simulink model "Assignment7"  (R2019a)
settings: Solver=FixedStepDiscrete  StartTime=0.0  StopTime=40  FixedStep=1  RelTol=1e-3
libraries: simulink x3
settings Model: Creator=Acer  LastModifiedBy=Acer

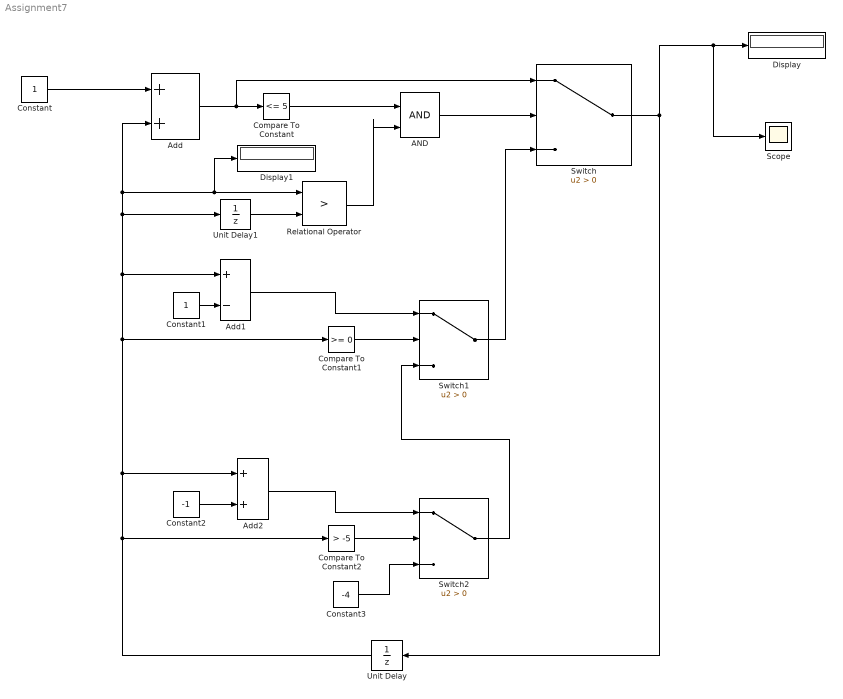
== system Assignment7 ==
  AND : Logic  IconShape=distinctive  AllPortsSameDT=off  OutDataTypeStr=boolean
  Add : Sum
  Add1 : Sum  Inputs=+-
  Add2 : Sum
  Compare To Constant : simulink/Logic and Bit Operations/Compare To Constant  relop=<=  const=5  OutDataTypeStr=boolean
  Compare To Constant1 : simulink/Logic and Bit Operations/Compare To Constant  relop=>=  const=0  OutDataTypeStr=boolean
  Compare To Constant2 : simulink/Logic and Bit Operations/Compare To Constant  relop=>  const=-5  OutDataTypeStr=boolean
  Constant : Constant
  Constant1 : Constant
  Constant2 : Constant  Value=-1
  Constant3 : Constant  Value=-4
  Display : Display
  Display1 : Display
  Relational Operator : RelationalOperator  Operator=>  OutDataTypeStr=boolean  RndMeth=Simplest
  Scope : Scope
  Switch : Switch  Criteria=u2 > Threshold
  Switch1 : Switch  Criteria=u2 > Threshold
  Switch2 : Switch  Criteria=u2 > Threshold
  Unit Delay : UnitDelay  InitialCondition=-1  SampleTime=-1  HasFrameUpgradeWarning=on
  Unit Delay1 : UnitDelay  InitialCondition=-2  SampleTime=-1  HasFrameUpgradeWarning=on
  wires:
  Constant/1 -> Add/1
  Add/1 -> Switch/1, Compare To Constant/1
  AND/1 -> Switch/2
  Compare To Constant/1 -> AND/1
  Switch/1 -> Scope/1, Display/1, Unit Delay/1
  Unit Delay/1 -> Add/2, Display1/1, Relational Operator/1, Unit Delay1/1, Add1/1, Compare To Constant1/1, Add2/1, Compare To Constant2/1
  Relational Operator/1 -> AND/2
  Unit Delay1/1 -> Relational Operator/2
  Compare To Constant1/1 -> Switch1/2
  Switch1/1 -> Switch/3
  Constant1/1 -> Add1/2
  Add1/1 -> Switch1/1
  Add2/1 -> Switch2/1
  Compare To Constant2/1 -> Switch2/2
  Constant2/1 -> Add2/2
  Constant3/1 -> Switch2/3
  Switch2/1 -> Switch1/3
